simulink model "motor_control"  (R2024b)
settings: Solver=VariableStepAuto  StartTime=0.0  StopTime=3  RelTol=1e-3
values from neighbouring files (symbols this model uses):
  K = 1.4    [runmotorcontrol.m]    (also in runmotorsimleft.m)
  kp = 3.5    [runmotorcontrol.m]
  sigma = 12    [runmotorcontrol.m]    (also in runmotorsimleft.m)
libraries: simulink x1
settings Model: Creator=iankeeffe  LastModifiedBy=iankeeffe

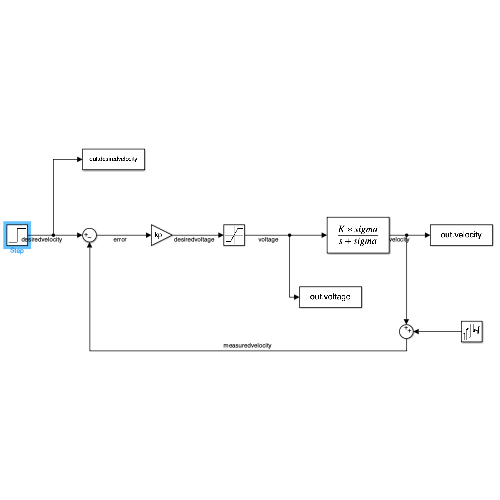
[thumbnail: Simulink's stored preview of the top-level diagram]
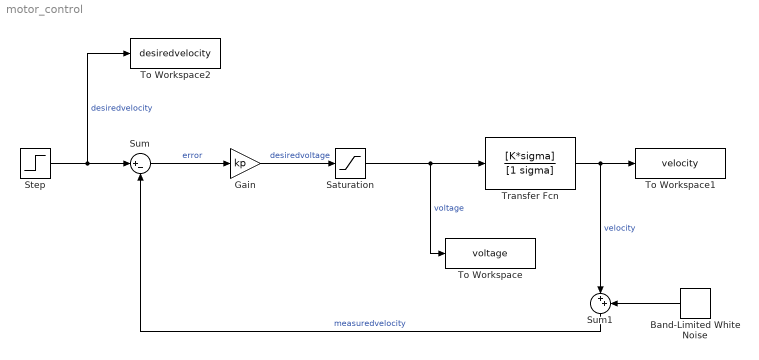
== system motor_control ==
  Band-Limited White Noise : simulink/Sources/Band-Limited White Noise  Cov=[0.0001]  Ts=0.01  seed=[23341]
  Gain : Gain  Gain=kp
  Saturation : Saturate  UpperLimit=7.5  LowerLimit=-7.5
  Step : Step  After=5  SampleTime=0
  Sum : Sum  Inputs=|+-
  Sum1 : Sum  Inputs=|++
  To Workspace : ToWorkspace  VariableName=voltage  SaveFormat=Timeseries  SampleTime=-1
  To Workspace1 : ToWorkspace  VariableName=velocity  SaveFormat=Timeseries  SampleTime=-1
  To Workspace2 : ToWorkspace  VariableName=desiredvelocity  SaveFormat=Timeseries  SampleTime=-1
  Transfer Fcn : TransferFcn  Numerator=[K*sigma]  Denominator=[1 sigma]
  wires:
  Saturation/1 -> To Workspace/1, Transfer Fcn/1  "voltage"
  Transfer Fcn/1 -> Sum1/1, To Workspace1/1  "velocity"
  Gain/1 -> Saturation/1  "desiredvoltage"
  Sum/1 -> Gain/1  "error"
  Step/1 -> To Workspace2/1, Sum/1  "desiredvelocity"
  Sum1/1 -> Sum/2  "measuredvelocity"
  Band-Limited White Noise/1 -> Sum1/2
